simulink library "sim_lib"  (R2022b)
settings: Solver=VariableStepAuto  StartTime=0.0  StopTime=10.0  RelTol=1e-3
libraries: Raptor_lib x17, simulink x2
settings Model: Creator=serga  LastModifiedBy=serga

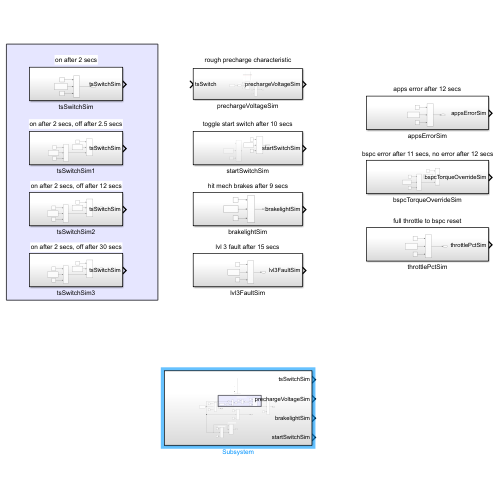
[thumbnail: Simulink's stored preview of the top-level diagram]
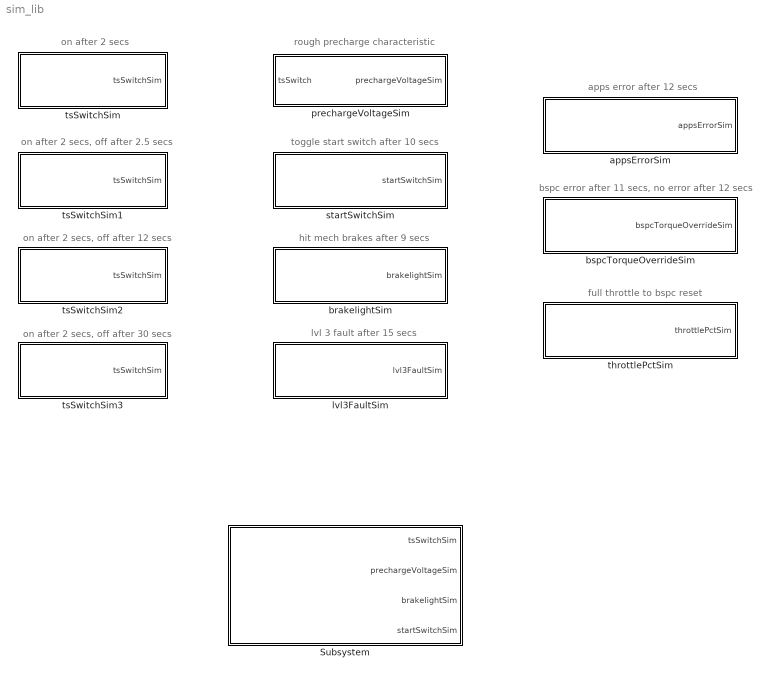
== system sim_lib ==
  note: apps error after 12 secs
  note: lvl 3 fault after 15 secs
  note: on after 2 secs, off after 30 secs
  note: hit mech brakes after 9 secs
  note: rough precharge characteristic
  note: toggle start switch after 10 secs
  note: on after 2 secs, off after 12 secs
  note: on after 2 secs, off after 2.5 secs
  note: on after 2 secs
  note: full throttle to bspc reset
  note: bspc error after 11 secs, no error after 12 secs
  Subsystem : Subsystem
  appsErrorSim : Subsystem
  brakelightSim : Subsystem
  bspcTorqueOverrideSim : Subsystem
  lvl3FaultSim : Subsystem
  prechargeVoltageSim : Subsystem
  startSwitchSim : Subsystem
  throttlePctSim : Subsystem
  tsSwitchSim : Subsystem
  tsSwitchSim1 : Subsystem
  tsSwitchSim2 : Subsystem
  tsSwitchSim3 : Subsystem

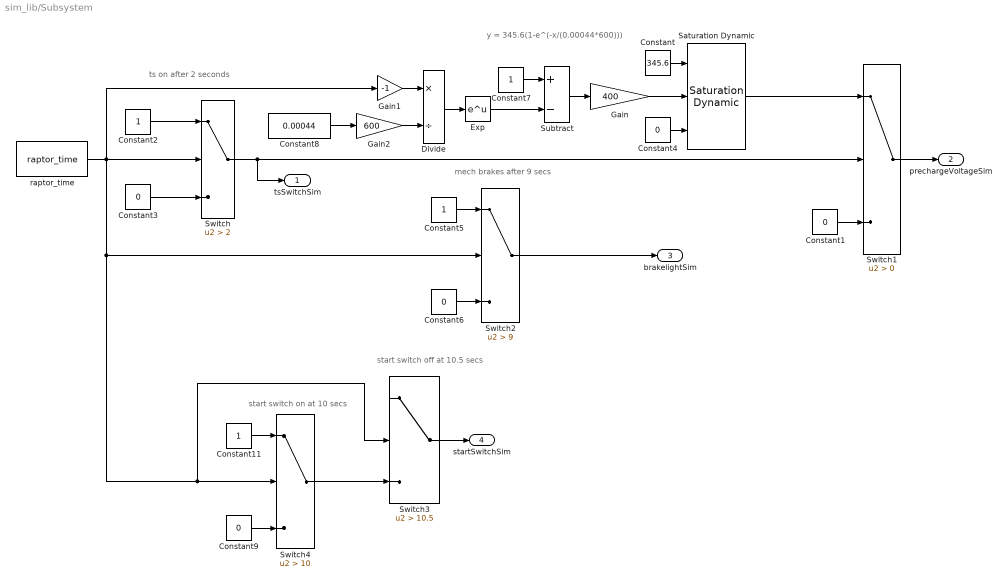
== system sim_lib/Subsystem ==
  note: start switch on at 10 secs
  note: start switch off at 10.5 secs
  note: y = 345.6(1-e^(-x/(0.00044*600)))
  note: mech brakes after 9 secs
  note: ts on after 2 seconds
  Constant : Constant  Value=345.6
  Constant{1,3..4,6,9} (5 alike) : Constant  Value=0
  Constant{2,5,7,11} (4 alike) : Constant
  Constant8 : Constant  Value=0.00044
  Divide : Product  Inputs=*/
  Exp : Math
  Gain : Gain  Gain=400
  Gain1 : Gain  Gain=-1
  Gain2 : Gain  Gain=600
  Saturation Dynamic : simulink/Discontinuities/Saturation Dynamic  OutMin=[]  OutMax=[]  OutDataTypeStr=Inherit: Same as second input  OutDataType=fixdt(1, 16)  OutScaling=2^-10  DoSatur=off
  Subtract : Sum  Inputs=+-
  Switch : Switch  Criteria=u2 > Threshold  Threshold=2  SaturateOnIntegerOverflow=off  InputSameDT=off
  Switch1 : Switch  Criteria=u2 > Threshold  SaturateOnIntegerOverflow=off  InputSameDT=off
  Switch2 : Switch  Criteria=u2 > Threshold  Threshold=9  SaturateOnIntegerOverflow=off  InputSameDT=off
  Switch3 : Switch  Criteria=u2 > Threshold  Threshold=10.5  SaturateOnIntegerOverflow=off  InputSameDT=off
  Switch4 : Switch  Criteria=u2 > Threshold  Threshold=10  SaturateOnIntegerOverflow=off  InputSameDT=off
  raptor_time : Raptor_lib/Triggers/raptor_time  unit=seconds
      settings: SourceProductName=Raptor
  tsSwitchSim : Outport
  prechargeVoltageSim : Outport  Port=2
  brakelightSim : Outport  Port=3
  startSwitchSim : Outport  Port=4
  wires:
  Constant3/1 -> Switch/3
  Constant2/1 -> Switch/1
  Switch1/1 -> prechargeVoltageSim/1
  Constant4/1 -> Saturation Dynamic/3
  Constant/1 -> Saturation Dynamic/1
  Switch/1 -> tsSwitchSim/1, Switch1/2
  Constant1/1 -> Switch1/3
  Constant6/1 -> Switch2/3
  Constant5/1 -> Switch2/1
  Switch2/1 -> brakelightSim/1
  Gain/1 -> Saturation Dynamic/2
  Constant7/1 -> Subtract/1
  Divide/1 -> Exp/1
  Constant8/1 -> Gain2/1
  Exp/1 -> Subtract/2
  Subtract/1 -> Gain/1
  Gain1/1 -> Divide/1
  Saturation Dynamic/1 -> Switch1/1
  Gain2/1 -> Divide/2
  Switch4/1 -> Switch3/3
  raptor_time/1 -> Gain1/1, Switch3/2, Switch4/2, Switch2/2, Switch/2
  Switch3/1 -> startSwitchSim/1
  Constant9/1 -> Switch4/3
  Constant11/1 -> Switch4/1

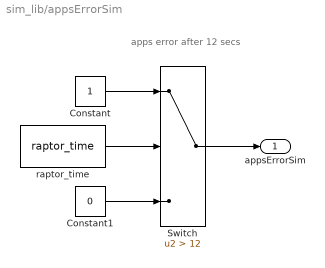
== system sim_lib/appsErrorSim ==
  note: apps error after 12 secs
  Constant : Constant
  Constant1 : Constant  Value=0
  Switch : Switch  Criteria=u2 > Threshold  Threshold=12  SaturateOnIntegerOverflow=off  InputSameDT=off
  raptor_time : Raptor_lib/Triggers/raptor_time  unit=seconds
      settings: SourceProductName=Raptor
  appsErrorSim : Outport
  wires:
  raptor_time/1 -> Switch/2
  Constant1/1 -> Switch/3
  Switch/1 -> appsErrorSim/1
  Constant/1 -> Switch/1

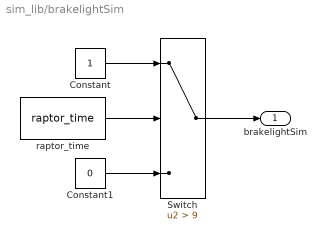
== system sim_lib/brakelightSim ==
  Constant : Constant
  Constant1 : Constant  Value=0
  Switch : Switch  Criteria=u2 > Threshold  Threshold=9  SaturateOnIntegerOverflow=off  InputSameDT=off
  raptor_time : Raptor_lib/Triggers/raptor_time  unit=seconds
      settings: SourceProductName=Raptor
  brakelightSim : Outport
  wires:
  Switch/1 -> brakelightSim/1
  Constant/1 -> Switch/1
  raptor_time/1 -> Switch/2
  Constant1/1 -> Switch/3

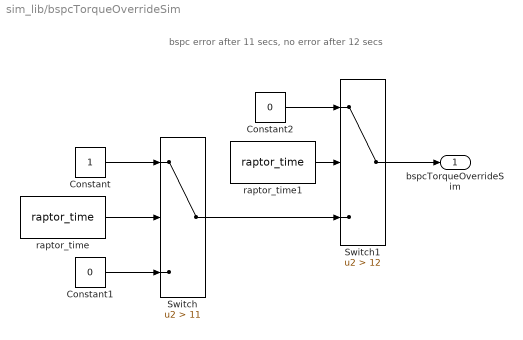
== system sim_lib/bspcTorqueOverrideSim ==
  note: bspc error after 11 secs, no error after 12 secs
  Constant : Constant
  Constant1 : Constant  Value=0
  Constant2 : Constant  Value=0
  Switch : Switch  Criteria=u2 > Threshold  Threshold=11  SaturateOnIntegerOverflow=off  InputSameDT=off
  Switch1 : Switch  Criteria=u2 > Threshold  Threshold=12  SaturateOnIntegerOverflow=off  InputSameDT=off
  raptor_time : Raptor_lib/Triggers/raptor_time  unit=seconds
      settings: SourceProductName=Raptor
  raptor_time1 : Raptor_lib/Triggers/raptor_time  unit=seconds
      settings: SourceProductName=Raptor
  bspcTorqueOverrideSim : Outport
  wires:
  raptor_time/1 -> Switch/2
  Constant/1 -> Switch/1
  Constant1/1 -> Switch/3
  Switch/1 -> Switch1/3
  raptor_time1/1 -> Switch1/2
  Switch1/1 -> bspcTorqueOverrideSim/1
  Constant2/1 -> Switch1/1

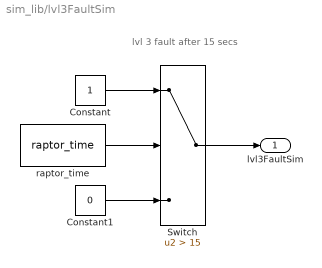
== system sim_lib/lvl3FaultSim ==
  note: lvl 3 fault after 15 secs
  Constant : Constant
  Constant1 : Constant  Value=0
  Switch : Switch  Criteria=u2 > Threshold  Threshold=15  SaturateOnIntegerOverflow=off  InputSameDT=off
  raptor_time : Raptor_lib/Triggers/raptor_time  unit=seconds
      settings: SourceProductName=Raptor
  lvl3FaultSim : Outport
  wires:
  raptor_time/1 -> Switch/2
  Constant/1 -> Switch/1
  Switch/1 -> lvl3FaultSim/1
  Constant1/1 -> Switch/3

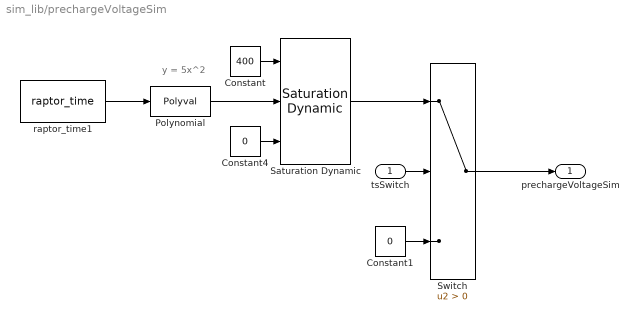
== system sim_lib/prechargeVoltageSim ==
  note: y = 5x^2
  tsSwitch : Inport
  Constant : Constant  Value=400
  Constant1 : Constant  Value=0
  Constant4 : Constant  Value=0
  Polynomial : Polyval  Coefs=[5, 0, 0]
  Saturation Dynamic : simulink/Discontinuities/Saturation Dynamic  OutMin=[]  OutMax=[]  OutDataTypeStr=Inherit: Same as second input  OutDataType=fixdt(1, 16)  OutScaling=2^-10  DoSatur=off
  Switch : Switch  Criteria=u2 > Threshold  SaturateOnIntegerOverflow=off  InputSameDT=off
  raptor_time1 : Raptor_lib/Triggers/raptor_time  unit=seconds
      settings: SourceProductName=Raptor
  prechargeVoltageSim : Outport
  wires:
  tsSwitch/1 -> Switch/2
  Saturation Dynamic/1 -> Switch/1
  Constant4/1 -> Saturation Dynamic/3
  raptor_time1/1 -> Polynomial/1
  Polynomial/1 -> Saturation Dynamic/2
  Constant/1 -> Saturation Dynamic/1
  Switch/1 -> prechargeVoltageSim/1
  Constant1/1 -> Switch/3

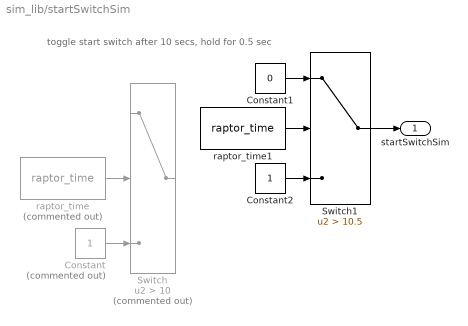
== system sim_lib/startSwitchSim ==
  note: toggle start switch after 10 secs, hold for 0.5 sec
  Constant : Constant  Commented=on
  Constant1 : Constant  Value=0
  Constant2 : Constant
  Switch : Switch  Commented=on  Criteria=u2 > Threshold  Threshold=10  SaturateOnIntegerOverflow=off  InputSameDT=off
  Switch1 : Switch  Criteria=u2 > Threshold  Threshold=10.5  SaturateOnIntegerOverflow=off  InputSameDT=off
  raptor_time : Raptor_lib/Triggers/raptor_time  Commented=on  unit=seconds
      settings: SourceProductName=Raptor
  raptor_time1 : Raptor_lib/Triggers/raptor_time  unit=seconds
      settings: SourceProductName=Raptor
  startSwitchSim : Outport
  wires:
  Constant/1 -> Switch/3
  raptor_time/1 -> Switch/2
  raptor_time1/1 -> Switch1/2
  Switch1/1 -> startSwitchSim/1
  Constant1/1 -> Switch1/1
  Constant2/1 -> Switch1/3

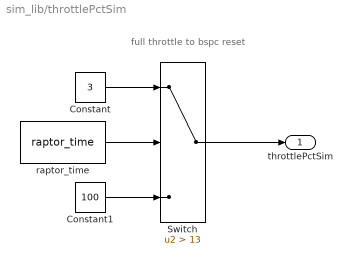
== system sim_lib/throttlePctSim ==
  note: full throttle to bspc reset
  Constant : Constant  Value=3
  Constant1 : Constant  Value=100
  Switch : Switch  Criteria=u2 > Threshold  Threshold=13  SaturateOnIntegerOverflow=off  InputSameDT=off
  raptor_time : Raptor_lib/Triggers/raptor_time  unit=seconds
      settings: SourceProductName=Raptor
  throttlePctSim : Outport
  wires:
  Constant/1 -> Switch/1
  Constant1/1 -> Switch/3
  Switch/1 -> throttlePctSim/1
  raptor_time/1 -> Switch/2

== system sim_lib/tsSwitchSim ==
  note: turn on after 2 seconds
  Constant2 : Constant
  Constant3 : Constant  Value=0
  Switch : Switch  Criteria=u2 > Threshold  Threshold=2  SaturateOnIntegerOverflow=off  InputSameDT=off
  raptor_time : Raptor_lib/Triggers/raptor_time  unit=seconds
      settings: SourceProductName=Raptor
  tsSwitchSim : Outport
  wires:
  Constant2/1 -> Switch/1
  raptor_time/1 -> Switch/2
  Constant3/1 -> Switch/3
  Switch/1 -> tsSwitchSim/1

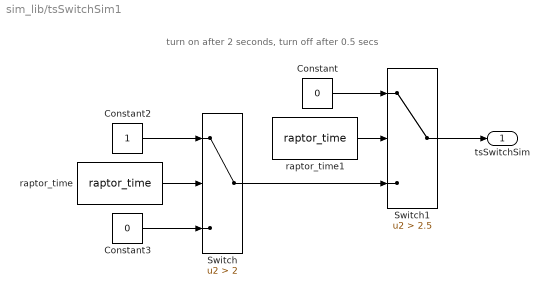
== system sim_lib/tsSwitchSim1 ==
  note: turn on after 2 seconds, turn off after 0.5 secs
  Constant : Constant  Value=0
  Constant2 : Constant
  Constant3 : Constant  Value=0
  Switch : Switch  Criteria=u2 > Threshold  Threshold=2  SaturateOnIntegerOverflow=off  InputSameDT=off
  Switch1 : Switch  Criteria=u2 > Threshold  Threshold=2.5  SaturateOnIntegerOverflow=off  InputSameDT=off
  raptor_time : Raptor_lib/Triggers/raptor_time  unit=seconds
      settings: SourceProductName=Raptor
  raptor_time1 : Raptor_lib/Triggers/raptor_time  unit=seconds
      settings: SourceProductName=Raptor
  tsSwitchSim : Outport
  wires:
  Constant3/1 -> Switch/3
  raptor_time/1 -> Switch/2
  Switch/1 -> Switch1/3
  Constant2/1 -> Switch/1
  raptor_time1/1 -> Switch1/2
  Constant/1 -> Switch1/1
  Switch1/1 -> tsSwitchSim/1

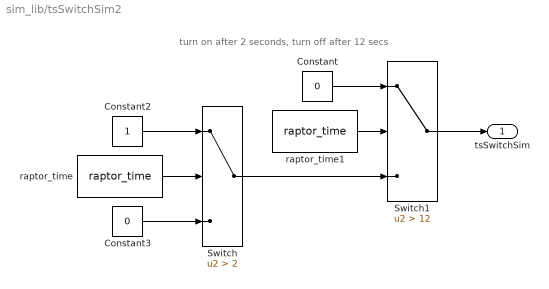
== system sim_lib/tsSwitchSim2 ==
  note: turn on after 2 seconds, turn off after 12 secs
  Constant : Constant  Value=0
  Constant2 : Constant
  Constant3 : Constant  Value=0
  Switch : Switch  Criteria=u2 > Threshold  Threshold=2  SaturateOnIntegerOverflow=off  InputSameDT=off
  Switch1 : Switch  Criteria=u2 > Threshold  Threshold=12  SaturateOnIntegerOverflow=off  InputSameDT=off
  raptor_time : Raptor_lib/Triggers/raptor_time  unit=seconds
      settings: SourceProductName=Raptor
  raptor_time1 : Raptor_lib/Triggers/raptor_time  unit=seconds
      settings: SourceProductName=Raptor
  tsSwitchSim : Outport
  wires:
  Constant2/1 -> Switch/1
  Switch/1 -> Switch1/3
  Constant3/1 -> Switch/3
  raptor_time/1 -> Switch/2
  Switch1/1 -> tsSwitchSim/1
  Constant/1 -> Switch1/1
  raptor_time1/1 -> Switch1/2

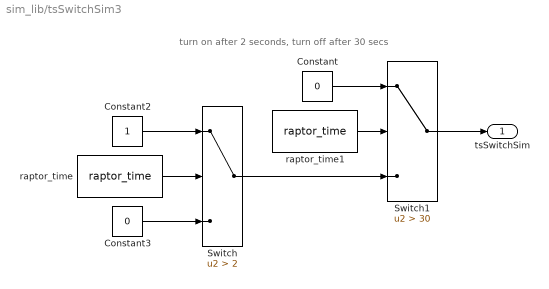
== system sim_lib/tsSwitchSim3 ==
  note: turn on after 2 seconds, turn off after 30 secs
  Constant : Constant  Value=0
  Constant2 : Constant
  Constant3 : Constant  Value=0
  Switch : Switch  Criteria=u2 > Threshold  Threshold=2  SaturateOnIntegerOverflow=off  InputSameDT=off
  Switch1 : Switch  Criteria=u2 > Threshold  Threshold=30  SaturateOnIntegerOverflow=off  InputSameDT=off
  raptor_time : Raptor_lib/Triggers/raptor_time  unit=seconds
      settings: SourceProductName=Raptor
  raptor_time1 : Raptor_lib/Triggers/raptor_time  unit=seconds
      settings: SourceProductName=Raptor
  tsSwitchSim : Outport
  wires:
  raptor_time/1 -> Switch/2
  Constant/1 -> Switch1/1
  Switch/1 -> Switch1/3
  Constant2/1 -> Switch/1
  Constant3/1 -> Switch/3
  raptor_time1/1 -> Switch1/2
  Switch1/1 -> tsSwitchSim/1
